simulink model "watervalve"  (R2023a)
settings: Solver=VariableStepAuto  StartTime=0.0  StopTime=10.0  RelTol=1e-3
settings Model: Creator=tiger  LastModifiedBy=tiger

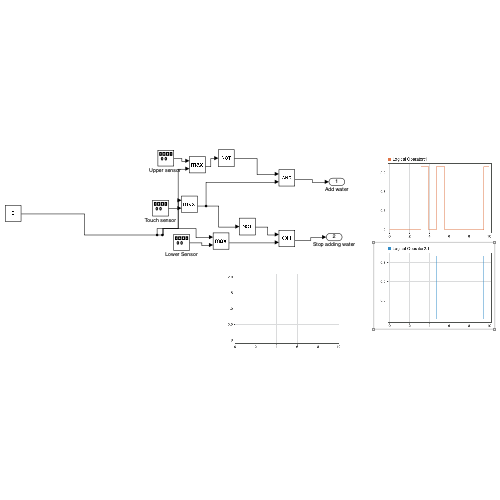
[thumbnail: Simulink's stored preview of the top-level diagram]
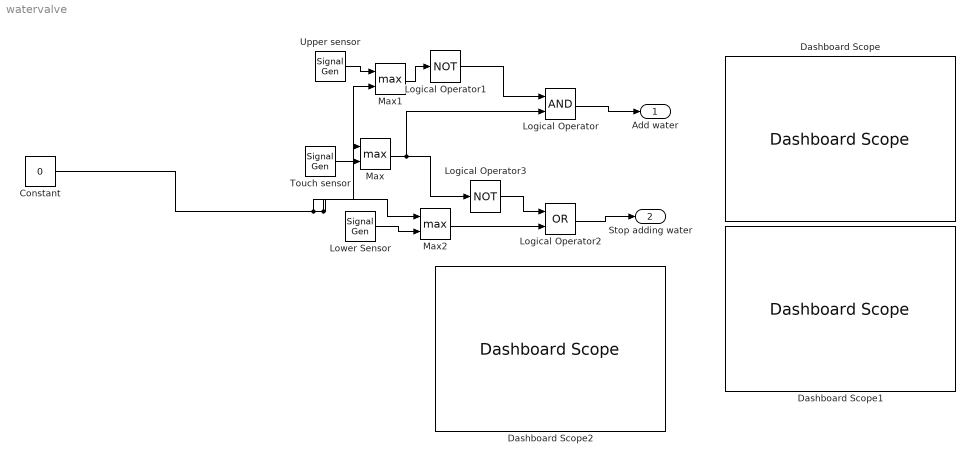
== system watervalve ==
  Constant : Constant  Value=0
  Dashboard Scope : DashboardScope
  Dashboard Scope1 : DashboardScope
  Dashboard Scope2 : DashboardScope
  Logical Operator : Logic  AllPortsSameDT=off  OutDataTypeStr=boolean
  Logical Operator1 : Logic  Operator=NOT  AllPortsSameDT=off  OutDataTypeStr=boolean
  Logical Operator2 : Logic  Operator=OR  AllPortsSameDT=off  OutDataTypeStr=boolean
  Logical Operator3 : Logic  Operator=NOT  AllPortsSameDT=off  OutDataTypeStr=boolean
  Lower Sensor : SignalGenerator  WaveForm=square  Frequency=2  Units=rad/sec
  Max : MinMax  Function=max  Inputs=2
  Max1 : MinMax  Function=max  Inputs=2
  Max2 : MinMax  Function=max  Inputs=2
  Touch sensor : SignalGenerator  WaveForm=square  Units=rad/sec
  "Upper sensor " : SignalGenerator  WaveForm=square  Frequency=4  Units=rad/sec
  Add water : Outport
  Stop adding water : Outport  Port=2
  wires:
  Logical Operator/1 -> Add water/1
  Logical Operator2/1 -> Stop adding water/1
  Logical Operator3/1 -> Logical Operator2/1
  Logical Operator1/1 -> Logical Operator/1
  Max2/1 -> Logical Operator2/2
  Touch sensor/1 -> Max/2
  Max/1 -> Logical Operator/2, Logical Operator3/1
  "Upper sensor "/1 -> Max1/1
  Max1/1 -> Logical Operator1/1
  Lower Sensor/1 -> Max2/2
  Constant/1 -> Max2/1, Max1/2, Max/1
